simulink model "Simulink"  (R2024b)
settings: Solver=VariableStepAuto  StartTime=0.0  StopTime=50  RelTol=1e-3
values from neighbouring files (symbols this model uses):
  K = acker(A, B, poles)    [Projekt_main.m]    (also in Projekt_mozg_egy.m)
  K0 = lqr(A,B,Q,R)    [masik_K.m]
settings Model: Creator=juhas  LastModifiedBy=juhas

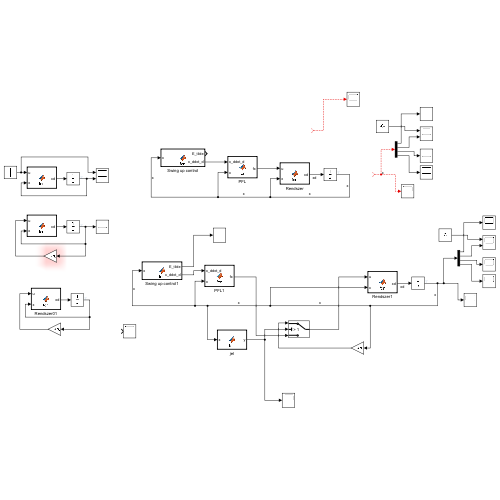
[thumbnail: Simulink's stored preview of the top-level diagram]
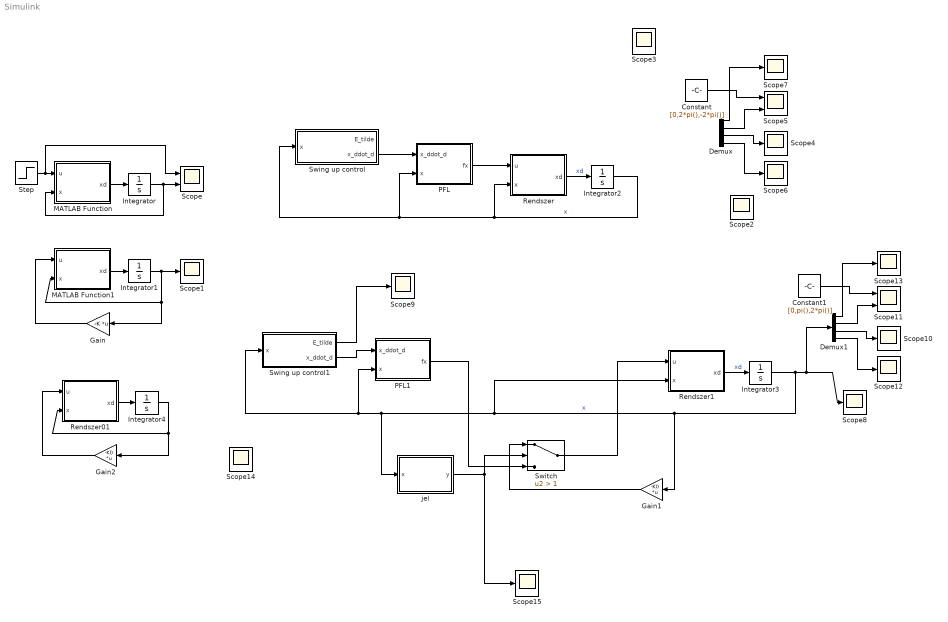
== system Simulink ==
  Constant : Constant  Value=[0,2*pi(),-2*pi()]
  Constant1 : Constant  Value=[0,pi(),2*pi()]
  Demux : Demux
  Demux1 : Demux
  Gain : Gain  Gain=-K  Multiplication=Matrix(K*u)
  Gain1 : Gain  Gain=-K0  Multiplication=Matrix(K*u)
  Gain2 : Gain  Gain=-K0  Multiplication=Matrix(K*u)
  Integrator : Integrator  InitialCondition=[0;pi();0;0]
  Integrator1 : Integrator  InitialCondition=[0;0.2;0;0]
  Integrator2 : Integrator  InitialCondition=[0;pi()+0.1;0;0]
  Integrator3 : Integrator  InitialCondition=[0;pi()+0.1;0;0]
  Integrator4 : Integrator  InitialCondition=[0;0.3;0;0]
  MATLAB Function : MATLAB Function  TreatAsAtomicUnit=on
  MATLAB Function1 : MATLAB Function  TreatAsAtomicUnit=on
  PFL : MATLAB Function  TreatAsAtomicUnit=on
  PFL1 : MATLAB Function  TreatAsAtomicUnit=on
  Rendszer : MATLAB Function  TreatAsAtomicUnit=on
  Rendszer01 : MATLAB Function  TreatAsAtomicUnit=on
  Rendszer1 : MATLAB Function  TreatAsAtomicUnit=on
  Scope : Scope  NumInputPorts=2
  Scope{1..4,6..10,12..15} (13 alike) : Scope
  Scope11 : Scope  NumInputPorts=2
  Scope5 : Scope  NumInputPorts=2
  Step : Step  Time=5  After=0.5  SampleTime=0
  Swing up control : MATLAB Function  TreatAsAtomicUnit=on
  Swing up control1 : MATLAB Function  TreatAsAtomicUnit=on
  Switch : Switch  Criteria=u2 > Threshold  Threshold=1  SaturateOnIntegerOverflow=off  InputSameDT=off
  jel : MATLAB Function  TreatAsAtomicUnit=on
  wires:
  MATLAB Function/1(xd) -> Integrator/1
  Integrator/1 -> Scope/2, MATLAB Function/2(x)
  Step/1 -> Scope/1, MATLAB Function/1(u)
  Gain/1 -> MATLAB Function1/1(u)
  MATLAB Function1/1(xd) -> Integrator1/1
  Integrator1/1 -> Scope1/1, Gain/1, MATLAB Function1/2(x)
  Rendszer/1(xd) -> Integrator2/1  "xd"
  PFL/1(fx) -> Rendszer/1(u)
  Swing up control/2(x_ddot_d) -> PFL/1(x_ddot_d)
  Integrator2/1 -> Swing up control/1(x), PFL/2(x), Rendszer/2(x)  "x"
  Constant1/1 -> Scope11/1
  Integrator3/1 -> jel/1(x), Swing up control1/1(x), PFL1/2(x), Rendszer1/2(x), Gain1/1, Demux1/1, Scope8/1  "x"
  Swing up control1/1(E_tilde) -> Scope9/1
  Swing up control1/2(x_ddot_d) -> PFL1/1(x_ddot_d)
  Demux1/3 -> Scope10/1
  Demux1/4 -> Scope12/1
  Demux1/2 -> Scope11/2
  Demux1/1 -> Scope13/1
  Rendszer1/1(xd) -> Integrator3/1  "xd"
  Integrator4/1 -> Gain2/1, Rendszer01/2(x)
  Rendszer01/1(xd) -> Integrator4/1
  Gain2/1 -> Rendszer01/1(u)
  Switch/1 -> Rendszer1/1(u)
  jel/1(y) -> Scope15/1, Switch/2
  PFL1/1(fx) -> Switch/3
  Gain1/1 -> Switch/1
  Demux/4 -> Scope6/1
  ? -> Demux/1, Scope2/1  "x"
  Demux/1 -> Scope7/1
  Constant/1 -> Scope5/1
  Demux/3 -> Scope4/1
  Demux/2 -> Scope5/2
  ? -> Scope3/1

== matlab function Simulink/MATLAB Function1 ==
  data: u input; x input; xd output
function xd = fcn(u, x)
g=9.81;
M=5;
m=0.3;
l=0.6;


phi=x(2);
phi_dot=x(4);
F=u;

xd1=x(3); %x_dot
xd2=x(4); %fi_dot
xd3=(2*l*m*sin(phi)*phi_dot^2 + 4*F - 3*g*m*cos(phi)*sin(phi))/(- 3*m*cos(phi)^2 + 4*M + 4*m);%x_ddot
xd4= - (3*(l*m*cos(phi)*sin(phi)*phi_dot^2 + 2*F*cos(phi) - 2*g*m*sin(phi) - 2*M*g*sin(phi)))/(l*(- 3*m*cos(phi)^2 + 4*M + 4*m));  %fi_ddot
xd=[xd1;xd2;xd3;xd4];

== matlab function Simulink/MATLAB Function ==
  data: u input; x input; xd output
function xd = fcn(u, x)
g=9.81;
M=2;
m=1;
l=1;

phi=x(2);
phi_dot=x(4);
F=u;

xd1=x(3); %x_dot
xd2=x(4); %fi_dot
xd3=(2*l*m*sin(phi)*phi_dot^2 + 4*F - 3*g*m*cos(phi)*sin(phi))/(- 3*m*cos(phi)^2 + 4*M + 4*m);%x_ddot
xd4= - (3*(l*m*cos(phi)*sin(phi)*phi_dot^2 + 2*F*cos(phi) - 2*g*m*sin(phi) - 2*M*g*sin(phi)))/(l*(- 3*m*cos(phi)^2 + 4*M + 4*m));  %fi_ddot
xd=[xd1;xd2;xd3;xd4];

== matlab function Simulink/Rendszer ==
  data: u input; x input; xd output
function xd = fcn(u, x)
g=9.81;
M=5;
m=0.3;
l=0.6;

phi=x(2);
phi_dot=x(4);
F=u;

xd1=x(3); %x_dot
xd2=x(4); %fi_dot
xd3=(2*l*m*sin(phi)*phi_dot^2 + 4*F - 3*g*m*cos(phi)*sin(phi))/(- 3*m*cos(phi)^2 + 4*M + 4*m);%x_ddot
xd4= -(3*(l*m*cos(phi)*sin(phi)*phi_dot^2 + 2*F*cos(phi) - 2*g*m*sin(phi) - 2*M*g*sin(phi)))/(l*(- 3*m*cos(phi)^2 + 4*M + 4*m));  %fi_ddot
xd=[xd1;xd2;xd3;xd4];

== matlab function Simulink/PFL ==
  data: x_ddot_d input; x input; fx output
function fx = fcn(x_ddot_d, x)
g=9.81;
M=5;
m=0.3;
l=0.6;

phi=x(2);
phi_dot=x(4);
fx=0.5*m*sin(phi)*(3*g*cos(phi)/2-l*phi_dot^2)+(M+m-3*m*cos(phi)/4)*x_ddot_d;

== matlab function Simulink/Swing up control ==
  data: E_tilde output; x input; x_ddot_d output
function [E_tilde,x_ddot_d] = fcn(x) %x az állapot vektor
phi=x(2);
phi_dot=x(4);

g=9.81;
M=5;
m=0.3;
l=0.6;


kE=5;  %erősítés k>0
kp=1;
kd=1;

c=3/4*m*l^2;
E_tilde=0.5*c*phi_dot^2+0.5*m*g*l*(cos(phi)-1);
x_ddot_d = kE*cos(phi)*phi_dot*E_tilde-kp*x(1)-kd*(3);

== matlab function Simulink/PFL1 ==
  data: x_ddot_d input; x input; fx output
function fx = fcn(x_ddot_d, x)
g=9.81;
M=5;
m=0.3;
l=0.6;
J=1;


phi=x(2);
phi_dot=x(4);
fx=(M+m-(m^2*l^2*cos(phi)^2)/(m*l^2+J))*x_ddot_d+(m^2*l^2*g*cos(phi)*sin(phi))/(m*l^2+J)-m*l*sin(phi)*phi_dot^2;

== matlab function Simulink/Rendszer1 ==
  data: u input; x input; xd output
function xd = fcn(u, x)
g=9.81;
M=5;
m=0.3;
l=0.6;
J=1;


phi=x(2);
phi_dot=x(4);
F=u;

xd1=x(3); %x_dot
xd2=x(4); %fi_dot
xd3=(sin(phi)*l^3*m^2*phi_dot^2 - g*cos(phi)*sin(phi)*l^2*m^2 + F*l^2*m + J*sin(phi)*l*m*phi_dot^2 + F*J)/(- l^2*m^2*cos(phi)^2 + l^2*m^2 + M*l^2*m + J*m + J*M);%x_ddot
xd4= -(l*m*(l*m*cos(phi)*sin(phi)*phi_dot^2 + F*cos(phi) - g*m*sin(phi) - M*g*sin(phi)))/(- l^2*m^2*cos(phi)^2 + l^2*m^2 + M*l^2*m + J*m + J*M);  %fi_ddot
xd=[xd1;xd2;xd3;xd4];

== matlab function Simulink/Swing up control1 ==
  data: E_tilde output; x input; x_ddot_d output
function [E_tilde,x_ddot_d] = fcn(x) %x az állapot vektor
phi=x(2);
phi_dot=x(4);

g=9.81;
M=5;
m=0.3;
l=0.6;


kE=1;  %erősítés k>0
kp=1.5;
kd=5;

c=3/4*m*l^2;
E_tilde=0.5*c*phi_dot^2+0.5*m*g*l*(cos(phi)-1);
x_ddot_d = -kE*cos(phi)*phi_dot*E_tilde-kp*x(1)-kd*(3);

== matlab function Simulink/Rendszer01 ==
  data: u input; x input; xd output
function xd = fcn(u, x)
g=9.81;
M=5;
m=0.3;
l=0.6;
J=1;


phi=x(2);
phi_dot=x(4);
F=u;

xd1=x(3); %x_dot
xd2=x(4); %fi_dot
xd3=(sin(phi)*l^3*m^2*phi_dot^2 - g*cos(phi)*sin(phi)*l^2*m^2 + F*l^2*m + J*sin(phi)*l*m*phi_dot^2 + F*J)/(- l^2*m^2*cos(phi)^2 + l^2*m^2 + M*l^2*m + J*m + J*M);%x_ddot
xd4= -(l*m*(l*m*cos(phi)*sin(phi)*phi_dot^2 + F*cos(phi) - g*m*sin(phi) - M*g*sin(phi)))/(- l^2*m^2*cos(phi)^2 + l^2*m^2 + M*l^2*m + J*m + J*M);  %fi_ddot
xd=[xd1;xd2;xd3;xd4];

== matlab function Simulink/jel ==
  data: x input; y output
function y = fcn(x)
phi=x(2);

if abs(phi-2*pi())<0.2
    y=2;
else
    y=0;
end
